simulink model "Without Saturation Simulink Model"  (R2018b)
settings: Solver=VariableStepAuto  StartTime=0.0  StopTime=100  RelTol=1e-3
libraries: simulink_extras x3, dspinverses x1, simulink x1
settings Model: Creator=sphillip  LastModifiedBy=sphillip
settings SFSimCC: SimUseLocalCustomCode=off
settings RTWCC: RTWUseLocalCustomCode=off

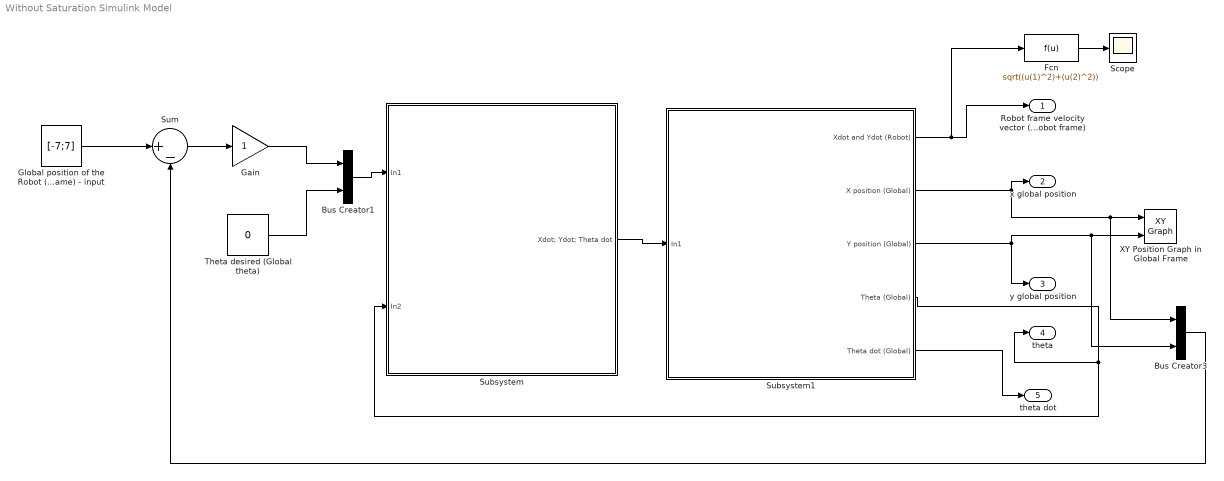
== system Without Saturation Simulink Model ==
  Bus Creator1 : BusCreator  Inputs=2
  Bus Creator3 : BusCreator  Inputs=2
  Fcn : Fcn  Expr=sqrt((u(1)^2)+(u(2)^2))
  Gain : Gain
  "Global position of the Robot (X, Y position of Global Frame) - input" : Constant  Value=[-7;7]
  Scope : Scope
  Subsystem : Subsystem
  Subsystem1 : Subsystem
  Sum : Sum  Inputs=|+-
  Theta desired (Global theta) : Constant  Value=0
  XY Position Graph in Global Frame : simulink/Sinks/XY Graph  xmin=-10  xmax=10  ymin=-10  ymax=10  st=0.3
  Robot frame velocity vector (X dot and Ydot of Robot frame) : Outport
  x global position : Outport  Port=2
  y global position : Outport  Port=3
  theta : Outport  Port=4
  theta dot : Outport  Port=5
  wires:
  Subsystem1/3(Y position (Global)) -> Bus Creator3/2, XY Position Graph in Global Frame/2, y global position/1
  Subsystem1/2(X position (Global)) -> x global position/1, Bus Creator3/1, XY Position Graph in Global Frame/1
  Subsystem1/4(Theta (Global)) -> Subsystem/2(In2), theta/1
  Subsystem/1(Xdot; Ydot; Theta dot) -> Subsystem1/1(In1)
  Subsystem1/1(Xdot and Ydot (Robot)) -> Robot frame velocity vector (X dot and Ydot of Robot frame)/1, Fcn/1
  Subsystem1/5(Theta dot (Global)) -> theta dot/1
  "Global position of the Robot (X, Y position of Global Frame) - input"/1 -> Sum/1
  Bus Creator3/1 -> Sum/2
  Sum/1 -> Gain/1
  Gain/1 -> Bus Creator1/1
  Theta desired (Global theta)/1 -> Bus Creator1/2
  Bus Creator1/1 -> Subsystem/1(In1)
  Fcn/1 -> Scope/1

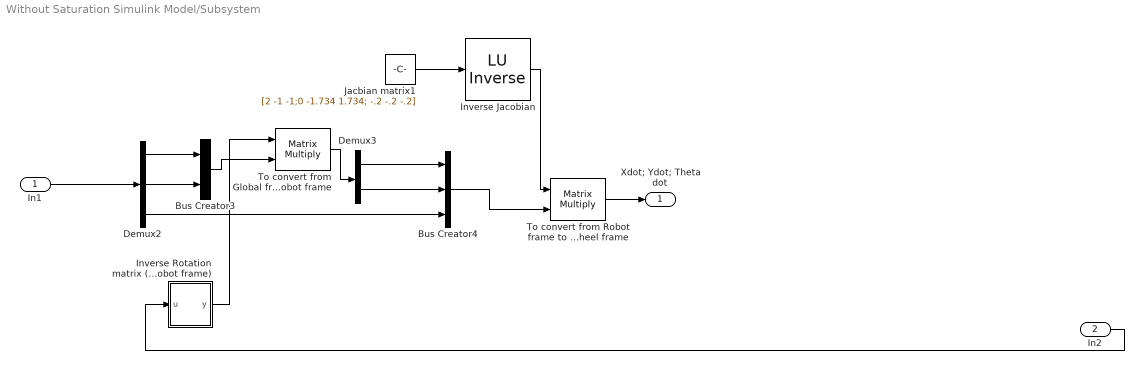
== system Without Saturation Simulink Model/Subsystem ==
  In1 : Inport
  In2 : Inport  Port=2
  Bus Creator3 : BusCreator  Inputs=2
  Bus Creator4 : BusCreator  Inputs=3
  Demux2 : Demux  Outputs=3
  Demux3 : Demux  Outputs=2
  Inverse Jacobian : dspinverses/ LU Inverse
      settings: SourceProductName=DSP System Toolbox
  Inverse Rotation matrix (used as a function to convert from Global frame to Robot frame) : MATLAB Function  TreatAsAtomicUnit=on
  Jacbian matrix1 : Constant  Value=[2 -1 -1;0 -1.734 1.734; -.2 -.2 -.2]  VectorParams1D=off
  To convert from Global frame to Robot frame : Product  Multiplication=Matrix(*)
  To convert from Robot frame to Wheel frame : Product  Multiplication=Matrix(*)
  Xdot; Ydot; Theta dot : Outport
  wires:
  Demux2/3 -> Bus Creator4/3
  To convert from Global frame to Robot frame/1 -> Demux3/1
  Inverse Rotation matrix (used as a function to convert from Global frame to Robot frame)/1(y) -> To convert from Global frame to Robot frame/1
  Inverse Jacobian/1 -> To convert from Robot frame to Wheel frame/1
  Jacbian matrix1/1 -> Inverse Jacobian/1
  To convert from Robot frame to Wheel frame/1 -> Xdot; Ydot; Theta dot/1
  In2/1 -> Inverse Rotation matrix (used as a function to convert from Global frame to Robot frame)/1(u)
  In1/1 -> Demux2/1
  Demux2/1 -> Bus Creator3/1
  Bus Creator3/1 -> To convert from Global frame to Robot frame/2
  Demux2/2 -> Bus Creator3/2
  Bus Creator4/1 -> To convert from Robot frame to Wheel frame/2
  Demux3/1 -> Bus Creator4/1
  Demux3/2 -> Bus Creator4/2

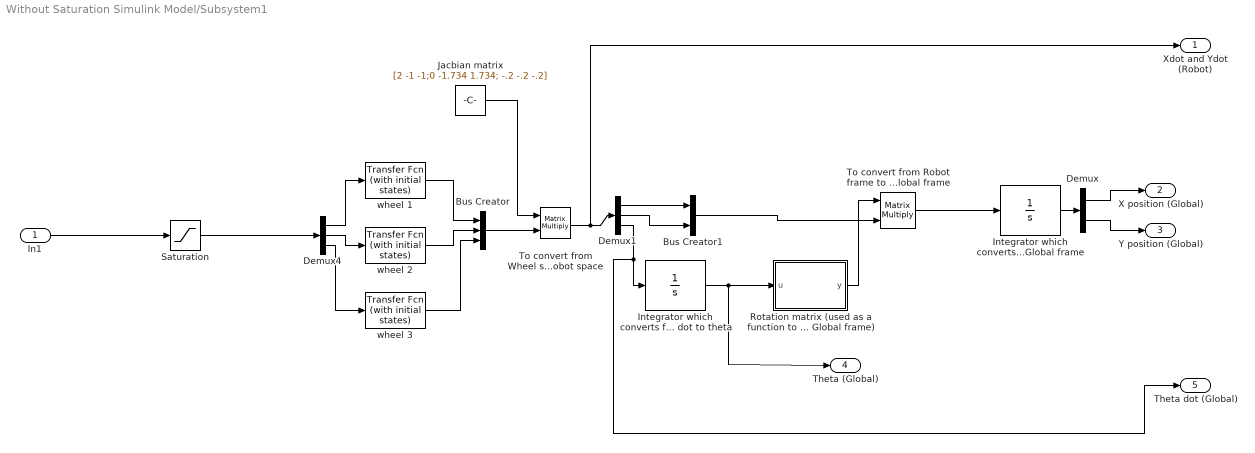
== system Without Saturation Simulink Model/Subsystem1 ==
  In1 : Inport
  Bus Creator : BusCreator  Inputs=3
  Bus Creator1 : BusCreator  Inputs=2
  Demux : Demux  Outputs=2
  Demux1 : Demux  Outputs=3
  Demux4 : Demux  Outputs=3
  "Integrator which converts from theta dot to theta " : Integrator
  "Integrator which converts from X and Y velocities (Xdot, Ydot) to X and Y positions of the Global frame " : Integrator
  Jacbian matrix : Constant  Value=[2 -1 -1;0 -1.734 1.734; -.2 -.2 -.2]  VectorParams1D=off
  Rotation matrix (used as a function to convert from Robot frame to Global frame) : MATLAB Function  TreatAsAtomicUnit=on
  Saturation : Saturate  UpperLimit=2*pi  LinearizeAsGain=off
  To convert from Robot frame to Global frame : Product  Multiplication=Matrix(*)
  To convert from Wheel space to Robot space : Product  Multiplication=Matrix(*)
  wheel 1 : simulink_extras/Additional Linear/Transfer Fcn (with initial states)  N=[1]  D="[1  1]"  X0=.5
  wheel 2 : simulink_extras/Additional Linear/Transfer Fcn (with initial states)  N=[1]  D="[1  1]"  X0=.5
  wheel 3 : simulink_extras/Additional Linear/Transfer Fcn (with initial states)  N=[1]  D="[1  1]"  X0=.5
  Xdot and Ydot (Robot) : Outport
  X position (Global) : Outport  Port=2
  Y position (Global) : Outport  Port=3
  Theta (Global) : Outport  Port=4
  Theta dot (Global) : Outport  Port=5
  wires:
  wheel 1/1 -> Bus Creator/1
  Demux4/2 -> wheel 2/1
  wheel 2/1 -> Bus Creator/2
  Demux1/1 -> Bus Creator1/1
  Demux/2 -> Y position (Global)/1
  To convert from Wheel space to Robot space/1 -> Xdot and Ydot (Robot)/1, Demux1/1
  Demux1/2 -> Bus Creator1/2
  "Integrator which converts from X and Y velocities (Xdot, Ydot) to X and Y positions of the Global frame "/1 -> Demux/1
  "Integrator which converts from theta dot to theta "/1 -> Theta (Global)/1, Rotation matrix (used as a function to convert from Robot frame to Global frame)/1(u)
  Rotation matrix (used as a function to convert from Robot frame to Global frame)/1(y) -> To convert from Robot frame to Global frame/1
  Bus Creator1/1 -> To convert from Robot frame to Global frame/2
  Jacbian matrix/1 -> To convert from Wheel space to Robot space/1
  Demux1/3 -> Theta dot (Global)/1, "Integrator which converts from theta dot to theta "/1
  Demux/1 -> X position (Global)/1
  Bus Creator/1 -> To convert from Wheel space to Robot space/2
  To convert from Robot frame to Global frame/1 -> "Integrator which converts from X and Y velocities (Xdot, Ydot) to X and Y positions of the Global frame "/1
  Demux4/1 -> wheel 1/1
  Demux4/3 -> wheel 3/1
  wheel 3/1 -> Bus Creator/3
  In1/1 -> Saturation/1
  Saturation/1 -> Demux4/1

== matlab function Without Saturation Simulink Model/Subsystem/Inverse Rotation matrix (used as a function to convert from Global frame to Robot frame) ==
  data: u input; y output
function y = fcn(u)
R = [cos(u) sin(u); -sin(u) cos(u)];
y = R;

== matlab function Without Saturation Simulink Model/Subsystem1/Rotation matrix (used as a function to convert from Robot frame to Global frame) ==
  data: u input; y output
function y = fcn(u)
R = [cos(u) -sin(u); sin(u) cos(u)];
y = R;
